simulink model "SimpleModel2"  (R2014a)
settings: Solver=ode3  StartTime=0.0  StopTime=tend  FixedStep=1e-3  MaxStep=0.1  RelTol=1e-3
values from neighbouring files (symbols this model uses):
  phi = -param_bar(2)/param_bar(1)    [test2D_data.m]    (also in test_tims_lambda_idea.m = [-param_bar(3)/param_bar(1), -param_bar(2)/param_bar(1) ])
settings Model: Creator=pjseiler  LastModifiedBy=MRDLAB
settings DataIOCC: SignalLoggingSaveFormat=ModelDataLogs
settings OptimizationCC: ExpressionDepthLimit=2147483647
settings DebuggingCC: UnderspecifiedInitializationDetection=Classic  MultiTaskDSMMsg=warning  MultiTaskCondExecSysMsg=none  FcnCallInpInsideContextMsg=EnableAllAsWarning  StateNameClashWarn=warning
settings RTWCC: IncludeERTFirstTime=on
settings GRTTargetCC: CombineOutputUpdateFcns=off  GRTInterface=on

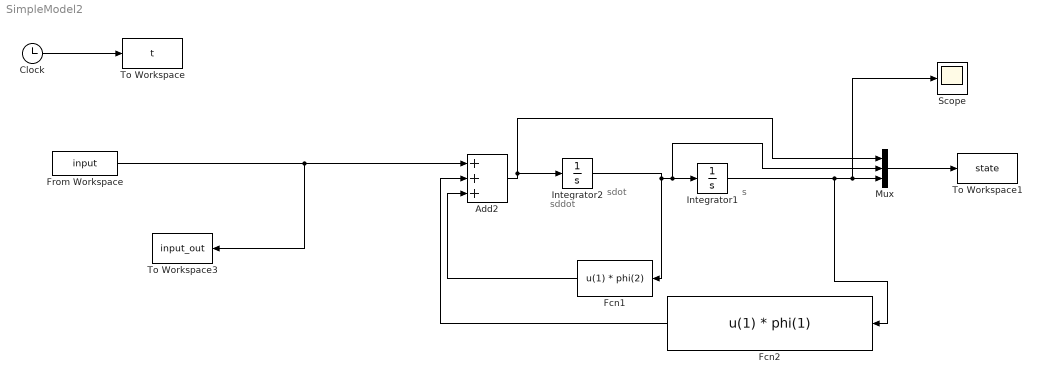
== system SimpleModel2 ==
  note: sddot
  note: sdot
  note: s
  Add2 : Sum  Inputs=+++
  Clock : Clock
  Fcn1 : Fcn  Expr=u(1) * phi(2)
  Fcn2 : Fcn  Expr=u(1) * phi(1)
  From Workspace : FromWorkspace  VariableName=input  SampleTime=0
  Integrator1 : Integrator
  Integrator2 : Integrator
  Mux : Mux  Inputs=3
  Scope : Scope
  To Workspace : ToWorkspace  VariableName=t  SampleTime=-1
  To Workspace1 : ToWorkspace  VariableName=state  SaveFormat=Timeseries  SampleTime=-1
  To Workspace3 : ToWorkspace  VariableName=input_out  SaveFormat=Timeseries  SampleTime=-1
  wires:
  Clock/1 -> To Workspace/1
  Integrator2/1 -> Fcn1/1, Integrator1/1, Mux/2
  Integrator1/1 -> Fcn2/1, Mux/3, Scope/1
  Add2/1 -> Integrator2/1, Mux/1
  Fcn1/1 -> Add2/3
  Fcn2/1 -> Add2/2
  Mux/1 -> To Workspace1/1
  From Workspace/1 -> Add2/1, To Workspace3/1
